simulink model "SimulinkLianxi"  (Simulink 9.1)
settings: Solver=VariableStepAuto  StartTime=0.0  StopTime=10.0  RelTol=1e-3
values from neighbouring files (symbols this model uses):
  A = [-0.0313 4.4879 0 -9.8;      -0.0058 -0.7458 0.9480 0;      -0.0002 -0.4479 -0.4609 0;      0        0       1       0]    [MoxingLianxi.m]
  B = [0.2063 -0.0516 -0.6532 0;      3.4847 -0.0561 0.0193 0]'    [MoxingLianxi.m]
  C = eye(4)    [MoxingLianxi.m]
  D = [0 0 0 0; 0 0 0 0]'    [MoxingLianxi.m]
settings Model: Creator=McQueen_Zero  LastModifiedBy=McQueen_Zero
settings DataIOCC: SaveFormat=Dataset
settings OptimizationCC: LifeSpan=auto
settings DebuggingCC: UnderspecifiedInitializationDetection=Simplified  MergeDetectMultiDrivingBlocksExec=error  SFUnexpectedBacktrackingDiag=error  SFNoUnconditionalDefaultTransitionDiag=error  SFExecutionAtInitializationDiag=warning
settings HardwareCC: ProdBitPerPointer=64  ProdBitPerSizeT=64  ProdBitPerPtrDiffT=64  ProdLargestAtomicFloat=Float  ProdIntDivRoundTo=Zero  ProdEndianess=LittleEndian  ProdWordSize=64  ProdHWDeviceType=Intel->x86-64 (Windows64)
settings ModelReferenceCC: PropagateSignalLabelsOutOfModel=on
settings CodeAppCC: StateflowObjectComments=off
settings GRTTargetCC: TargetLangStandard=C99 (ISO)  CombineOutputUpdateFcns=on  GRTInterface=off
settings ConfigComp: CovMetricSettings=dwe  CovHtmlReporting=off  CovSaveCumulativeToWorkspaceVar=off  CovSaveSingleToWorkspaceVar=off  CovExternalEMLEnable=on

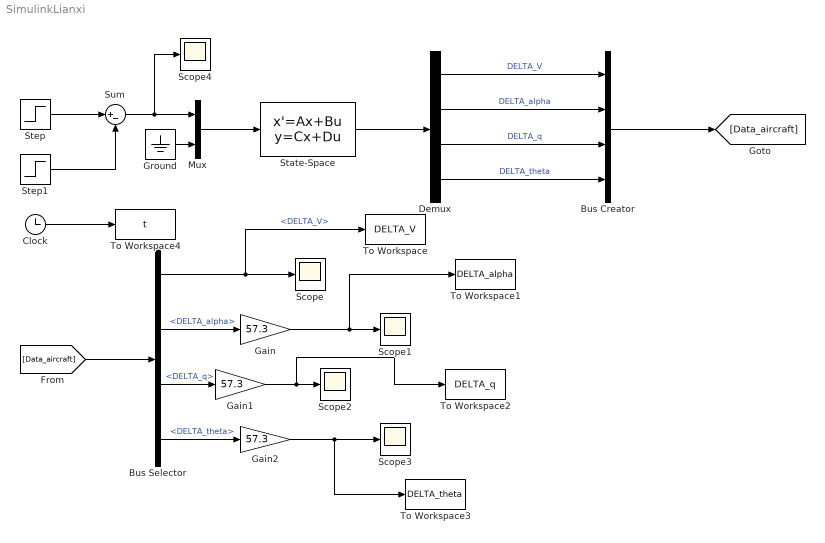
== system SimulinkLianxi ==
  Bus Creator : BusCreator  Inputs=4
  Bus Selector : BusSelector  OutputSignals=DELTA_V,DELTA_alpha,DELTA_q,DELTA_theta
  Clock : Clock
  Demux : Demux
  Gain : Gain  Gain=57.3
  Gain1 : Gain  Gain=57.3
  Gain2 : Gain  Gain=57.3
  Ground : Ground
  Mux : Mux  Inputs=2
  Scope{,1..4} (5 alike) : Scope
  State-Space : StateSpace  A=A  B=B  C=C  D=D  InitialCondition=0
  Step : Step  Time=0  After=5/57.3  SampleTime=0
  Step1 : Step  After=5/57.3  SampleTime=0
  Sum : Sum  Inputs=|+-
  To Workspace : ToWorkspace  VariableName=DELTA_V  SaveFormat=Timeseries  SampleTime=-1
  To Workspace1 : ToWorkspace  VariableName=DELTA_alpha  SaveFormat=Timeseries  SampleTime=-1
  To Workspace2 : ToWorkspace  VariableName=DELTA_q  SaveFormat=Timeseries  SampleTime=-1
  To Workspace3 : ToWorkspace  VariableName=DELTA_theta  SaveFormat=Timeseries  SampleTime=-1
  To Workspace4 : ToWorkspace  VariableName=t  SaveFormat=Timeseries  SampleTime=-1
  wires:
  Mux/1 -> State-Space/1
  Ground/1 -> Mux/2
  Sum/1 -> Mux/1, Scope4/1
  Step/1 -> Sum/1
  Step1/1 -> Sum/2
  State-Space/1 -> Demux/1
  Demux/1 -> Bus Creator/1  "DELTA_V"
  Demux/2 -> Bus Creator/2  "DELTA_alpha"
  Demux/3 -> Bus Creator/3  "DELTA_q"
  Demux/4 -> Bus Creator/4  "DELTA_theta"
  Bus Creator/1 -> [Data_aircraft]
  [Data_aircraft] -> Bus Selector/1
  Bus Selector/1 -> To Workspace/1, Scope/1  "<DELTA_V>"
  Bus Selector/3 -> Gain1/1  "<DELTA_q>"
  Bus Selector/2 -> Gain/1  "<DELTA_alpha>"
  Bus Selector/4 -> Gain2/1  "<DELTA_theta>"
  Gain1/1 -> To Workspace2/1, Scope2/1
  Gain/1 -> To Workspace1/1, Scope1/1
  Gain2/1 -> To Workspace3/1, Scope3/1
  Clock/1 -> To Workspace4/1
